simulink model "CloseLoop"  (R2024b)
settings: Solver=VariableStepAuto  StartTime=0.0  StopTime=10.0  FixedStep=0.001  RelTol=1e-7
values from neighbouring files (symbols this model uses):
  A = [0 0 0 1 0 0; 0 0 0 0 1 0; 0 0 0 0 0 1; 0 0 0 0 0 0; 0 0 0 0 0 0; 0 0 0 0 0 0]    [DefinedParameters.m]
  B = [0; 0; 0; 1; 1; 1]    [DefinedParameters.m]
  d = 0.0085    [DefinedParameters.m]
  D = J    (= 1.062e-08)    [DefinedParameters.m]
  Do = 0.0001    [DefinedParameters.m]
  F = 0.94    [DefinedParameters.m]
  g = 9.81    [DefinedParameters.m]
  h = 0.00515    [DefinedParameters.m]
  k = 71    [DefinedParameters.m]
  l = 0.03    [DefinedParameters.m]
  m = 0.0000354    (= 3.54e-05)    [DefinedParameters.m]
  r = 0.00485    [DefinedParameters.m]
libraries: simulink x12, matrix_library x2, slpidlib x1

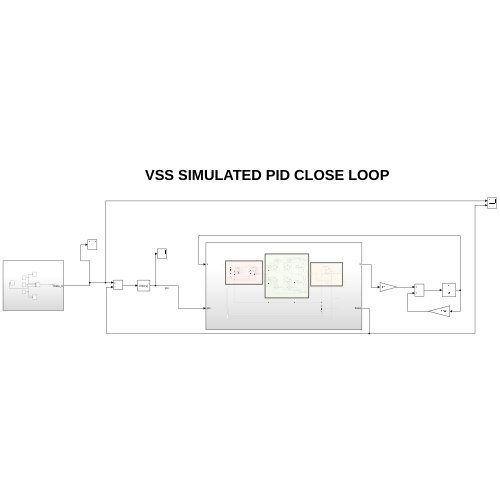
[thumbnail: Simulink's stored preview of the top-level diagram]
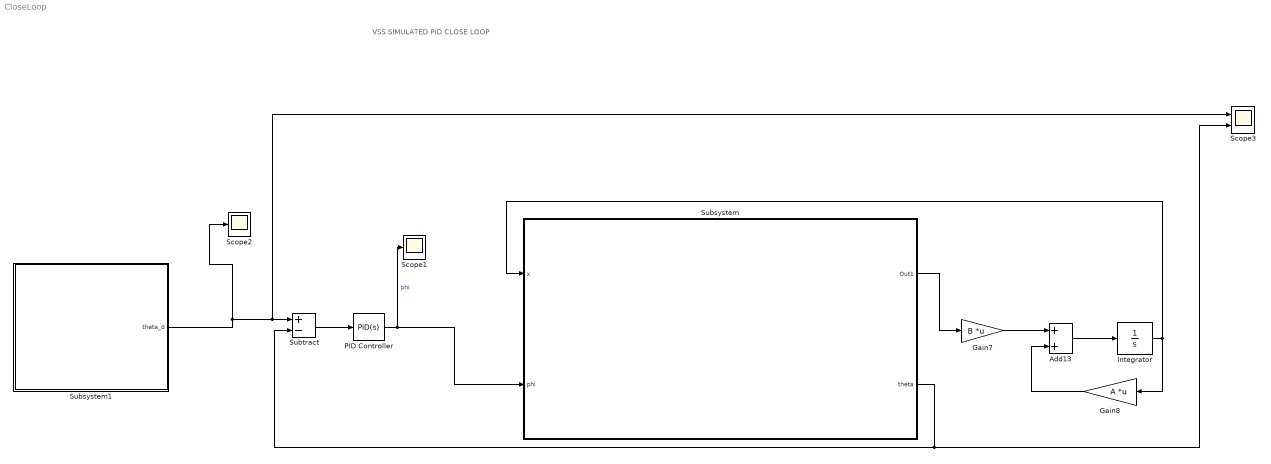
== system CloseLoop ==
  note: VSS SIMULATED PID CLOSE LOOP
  Add13 : Sum
  Gain7 : Gain  Gain=B  Multiplication=Matrix(K*u)
  Gain8 : Gain  Gain=A  Multiplication=Matrix(K*u)
  Integrator : Integrator  InitialCondition=[0;0;-1.6;0;0;0]
  PID Controller : slpidlib/PID Controller  Controller=PID  Form=Parallel  TimeDomain=Continuous-time  UseExternalTs=off  SampleTime=-1  IntegratorMethod=Forward Euler  FilterMethod=Forward Euler  ControllerParametersSource=internal  P=1  I=1.6  UseKiTs=off  D=0.5  UseExternalDerivativeSource=off  N=0  UseFilter=on  TunerSelectOption=Transfer Function Based (PID Tuner App)  InitialConditionSource=internal  InitialConditionForIntegrator=-1.7  InitialConditionForFilter=0  DifferentiatorICPrevScaledInput=0  ExternalReset=none  TrackingMode=off  Kt=1  LimitOutput=off  SatLimitsSource=internal  UpperSaturationLimit=inf  LowerSaturationLimit=-inf  LinearizeAsGain=on  AntiWindupMode=none  Kb=1  LimitIntegrator=off  UpperIntegratorSaturationLimit=inf  LowerIntegratorSaturationLimit=-inf  POutMin=[]  POutMax=[]  IOutMin=[]  IOutMax=[]  DOutMin=[]  DOutMax=[]  NOutMin=[]  NOutMax=[]  SumOutMin=[]  SumOutMax=[]  SaturationOutMin=[]  SaturationOutMax=[]  PParamMin=[]  PParamMax=[]  IParamMin=[]  IParamMax=[]  DParamMin=[]  DParamMax=[]  NParamMin=[]  NParamMax=[]  KbParamMin=[]  KbParamMax=[]  KtParamMin=[]  KtParamMax=[]  KbOutMin=[]  KbOutMax=[]  KtOutMin=[]  KtOutMax=[]  IntegratorOutMin=[]  IntegratorOutMax=[]  FilterOutMin=[]  FilterOutMax=[]  SumI1OutMin=[]  SumI1OutMax=[]  SumI2OutMin=[]  SumI2OutMax=[]  SumI3OutMin=[]  SumI3OutMax=[]  SumI4OutMin=[]  SumI4OutMax=[]  SumDOutMin=[]  SumDOutMax=[]  DifferentiatorOutMin=[]  DifferentiatorOutMax=[]  FilterDiffOutCoefMin=[]  FilterDiffOutCoefMax=[]  ReciprocalOutMin=[]  ReciprocalOutMax=[]  SumDenOutMin=[]  SumDenOutMax=[]  SumNumOutMin=[]  SumNumOutMax=[]  DivideOutMin=[]  DivideOutMax=[]  UdiffTsProdOutMin=[]  UdiffTsProdOutMax=[]  NTsProdOutMin=[]  NTsProdOutMax=[]  UintegralTsProdOutMin=[]  UintegralTsProdOutMax=[]  UngainTsProdOutMin=[]  UngainTsProdOutMax=[]  ClampingZeroOutDataTypeStr=Inherit: Inherit via back propagation  ClampingZeroOutMin=[]  ClampingZeroOutMax=[]  FilterDenConstantOutDataTypeStr=Inherit: Inherit via back propagation  FilterDenConstantOutMin=[]  FilterDenConstantOutMax=[]  PCopyOutDataTypeStr=Inherit: Inherit via back propagation  PCopyOutMin=[]  PCopyOutMax=[]  NCopyOutDataTypeStr=Inherit: Inherit via back propagation  NCopyOutMin=[]  NCopyOutMax=[]  IntegratorContinuousStateAttributes=''  IntegratorStateMustResolveToSignalObject=off  IntegratorRTWStateStorageClass=Auto  FilterContinuousStateAttributes=''  FilterStateMustResolveToSignalObject=off  FilterRTWStateStorageClass=Auto  ParallelPVariant=InternalParameters  IdealPVariant=Disabled  IVariant=InternalParameters  DVariant=InternalParameters  IntegratorVariant=Continuous  SatVariant=Disabled  AWVariant=Passthrough  PCopyVariant=Disabled  TRVariant=Disabled  FdbkBlocksVariant=Forward  IdealPFdbkVariant=Disabled  SatFdbkVariant=Disabled  DerivativeFilterVariant=ContFilter  NVariant=InternalParameters  NCopyVariant=Disabled  FilterICVariant=InternalICsFilter  IntegratorICVariant=InternalICs  ExternalResetVariant=Disabled  TRSumVariant=Passthrough  SumFdbkVariant=Disabled  SumVariant=Sum_PID  TsampFilterVariant=InternalTs  TsampNgainVariant=Passthrough  TsampIntegralVariant=Disabled_SignalSpec  ExternalSaturationOutDataTypeStr=Inherit: Same as second input  DerivativeSourceVariant=ErrorSignal  PreIntVariant=InternalPreInt
  Scope1 : Scope
  Scope2 : Scope
  Scope3 : Scope  NumInputPorts=2
  Subsystem : Subsystem
  Subsystem1 : Subsystem
  Subtract : Sum  Inputs=+-
  wires:
  Subtract/1 -> PID Controller/1
  Subsystem1/1(theta_d) -> Scope3/1, Subtract/1, Scope2/1
  PID Controller/1 -> Scope1/1, Subsystem/2(phi)  "phi"
  Subsystem/1(Out1) -> Gain7/1
  Gain8/1 -> Add13/2
  Integrator/1 -> Subsystem/1(x), Gain8/1
  Add13/1 -> Integrator/1
  Gain7/1 -> Add13/1
  Subsystem/2(theta) -> Subtract/2, Scope3/2

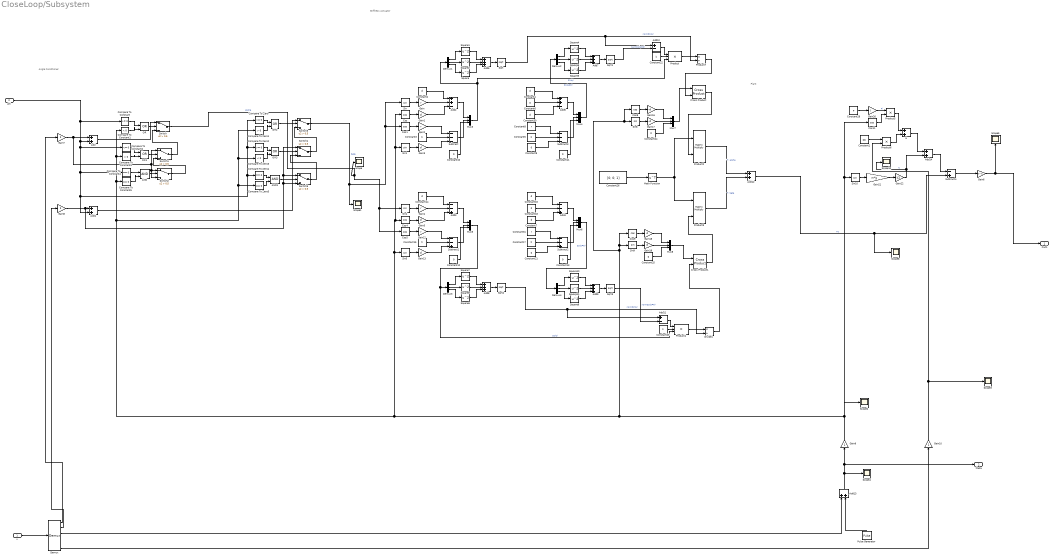
== system CloseLoop/Subsystem ==
  note: Plant
  note: Stiffness Actuator
  note: Angle Conditioner
  x : Inport
  phi : Inport  Port=2
  AND : Logic  IconShape=distinctive  AllPortsSameDT=off  OutDataTypeStr=boolean
  AND1 : Logic  IconShape=distinctive  AllPortsSameDT=off  OutDataTypeStr=boolean
  Add{,1,12..14} (5 alike) : Sum
  Add10 : Sum  Inputs=+-
  Add11 : Sum  Inputs=+-
  Add2 : Sum  Inputs=++-
  Add3 : Sum  Inputs=--+
  Add4 : Sum  Inputs=--+
  Add5 : Sum  Inputs=++-
  Add{6..9} (4 alike) : Sum  Inputs=+++
  Compare To Constant : simulink/Logic and Bit Operations/Compare To Constant  relop=>=  const=0  OutDataTypeStr=boolean
  Compare To Constant1 : simulink/Logic and Bit Operations/Compare To Constant  relop=<  const=0  OutDataTypeStr=boolean
  Compare To Constant2 : simulink/Logic and Bit Operations/Compare To Constant  relop=<=  const=0  OutDataTypeStr=boolean
  Compare To Constant3 : simulink/Logic and Bit Operations/Compare To Constant  relop=>  const=0  OutDataTypeStr=boolean
  Compare To Constant4 : simulink/Logic and Bit Operations/Compare To Constant  relop===  const=0  OutDataTypeStr=boolean
  Compare To Constant5 : simulink/Logic and Bit Operations/Compare To Constant  relop===  const=0  OutDataTypeStr=boolean
  Compare To Zero : simulink/Logic and Bit Operations/Compare To Zero  relop=<=  OutDataTypeStr=boolean
  Compare To Zero1 : simulink/Logic and Bit Operations/Compare To Zero  relop=>  OutDataTypeStr=boolean
  Compare To Zero2 : simulink/Logic and Bit Operations/Compare To Zero  relop=>=  OutDataTypeStr=boolean
  Compare To Zero3 : simulink/Logic and Bit Operations/Compare To Zero  relop=<  OutDataTypeStr=boolean
  Compare To Zero4 : simulink/Logic and Bit Operations/Compare To Zero  relop===  OutDataTypeStr=boolean
  Compare To Zero5 : simulink/Logic and Bit Operations/Compare To Zero  relop===  OutDataTypeStr=boolean
  Constant1 : Constant  Value=Do
  Constant{6,9..13,18,21,24..25} (10 alike) : Constant  Value=0
  Constant{2,4,7,14,16,30} (6 alike) : Constant  Value=d
  Constant{3,5,15,17} (4 alike) : Constant  Value=h
  Constant22 : Constant  Value=k
  Constant23 : Constant  Value=k
  Constant26 : Constant  Value=[0; 0; 1]
  Constant28 : Constant  Value=F
  Constant31 : Constant  Value=r
  Constant8 : Constant  Value=r
  Cos{,1,4..5,8..9,11} (7 alike) : Trigonometry  Operator=cos
  Cross Product : matrix_library/Cross Product
  Cross Product1 : matrix_library/Cross Product
  Demux : Demux  Outputs=6
  Demux{1..4} (4 alike) : Demux  Outputs=3
  Divide1 : Product  Inputs=*/
  Gain{,2,4,12} (4 alike) : Gain  Gain=r
  Gain{1,3,5,13,18..19} (6 alike) : Gain  Gain=d
  Gain{7..10} (4 alike) : Gain
  Gain16 : Gain  Gain=-d
  Gain17 : Gain  Gain=-d
  Gain21 : Gain  Gain=m*g
  Gain22 : Gain  Gain=l/2
  Gain26 : Gain  Gain=l
  Gain6 : Gain  Gain=D^-1
  H : Sum
  Math Function : Math  Operator=transpose
  Mux{3..8} (6 alike) : Mux  Inputs=3
  OR{,1..3} (4 alike) : Logic  Operator=OR  IconShape=distinctive  AllPortsSameDT=off  OutDataTypeStr=boolean
  Product : Product  Inputs=3
  Product1 : Product  Inputs=3
  Product2 : Product  Multiplication=Matrix(*)
  Product3 : Product  Multiplication=Matrix(*)
  Product5 : Product
  Product6 : Product
  Product7 : Product  Inputs=*/
  Pulse Generator : DiscretePulseGenerator  PulseType=Time based  Amplitude=0.02  Period=2.5  PulseWidth=0.5
  Scope{,1..5,8,10} (8 alike) : Scope
  Sin{,1,4..5,8..10} (7 alike) : Trigonometry
  Sqrt{,1..3} (4 alike) : Sqrt
  Square{,1..11} (12 alike) : Math  Operator=square
  Subtract : Sum  Inputs=---
  Subtract1 : Sum  Inputs=--+
  Subtract2 : Sum  Inputs=--+
  Subtract3 : Sum  Inputs=---
  Subtract4 : Sum  Inputs=-+
  Switch{,1..5} (6 alike) : Switch  Criteria=u2 > Threshold  Threshold=0.5  SaturateOnIntegerOverflow=off  InputSameDT=off
  Out1 : Outport
  theta : Outport  Port=2
  wires:
  x/1 -> Demux/1
  AND1/1 -> Switch5/2
  Switch5/1 -> Switch4/3
  Switch4/1 -> Switch3/3
  Add1/1 -> Switch3/1
  Gain8/1 -> Switch5/1, Switch4/1, Switch5/3, Add1/1
  Add/1 -> Switch/1
  Gain7/1 -> Add/1, Switch1/1, Switch2/3, Switch2/1
  OR3/1 -> Switch4/2
  OR2/1 -> Switch3/2
  Compare To Zero5/1 -> AND1/2
  Compare To Zero4/1 -> AND1/1
  Compare To Zero3/1 -> OR3/2
  Compare To Zero2/1 -> OR3/1
  Compare To Zero1/1 -> OR2/2
  Compare To Zero/1 -> OR2/1
  Switch2/1 -> Switch1/3
  AND/1 -> Switch2/2
  Compare To Constant5/1 -> AND/2
  Compare To Constant4/1 -> AND/1
  Constant16/1 -> Add4/1
  Sqrt3/1 -> Add11/2  "normS2(q=0)"
  Gain22/1 -> Scope10/1, Add14/2  "C"
  Product/1 -> Product7/1
  Switch/1 -> Scope/1, Sin4/1, Cos5/1  "alpha"
  Mux8/1 -> Cross Product1/1
  Gain4/1 -> Add3/2
  Add14/1 -> Subtract4/1
  Gain/1 -> Add2/2
  Demux3/3 -> Square6/1
  Product6/1 -> H/2
  Sin5/1 -> Gain13/1
  Math Function/1 -> Product3/1, Product2/1
  Cos11/1 -> Product5/2
  Product1/1 -> Divide1/1
  Add8/1 -> Sqrt2/1
  Constant6/1 -> Add5/2
  Constant21/1 -> Subtract2/3
  Constant26/1 -> Math Function/1
  Compare To Constant/1 -> OR/1
  Cos/1 -> Gain1/1
  Constant31/1 -> Subtract2/1
  Product3/1 -> Add12/2  "T, beta"
  Constant4/1 -> Add5/1
  Constant2/1 -> Add2/1
  Product2/1 -> Add12/1  "T, alpha"
  Subtract/1 -> Mux3/2
  Product5/1 -> H/1
  H/1 -> Add14/1
  Demux2/2 -> Square5/1
  Sin10/1 -> Gain21/1
  Gain1/1 -> Add2/3
  Cross Product1/1 -> Product3/2
  Mux6/1 -> Demux4/1  "S2(q=0)"
  Constant13/1 -> Mux6/3
  Demux3/1 -> Square7/1
  Constant22/1 -> Product/2
  Demux3/2 -> Square8/1
  Mux7/1 -> Cross Product/1
  Constant8/1 -> Subtract3/1
  Switch3/1 -> Scope1/1, Sin/1, Cos1/1  "beta"
  Cos5/1 -> Gain12/1
  Subtract1/1 -> Mux5/2
  Square8/1 -> Add8/2
  Gain13/1 -> Subtract1/3
  Cos9/1 -> Gain18/1
  Add11/1 -> Product1/1
  Square1/1 -> Add6/1
  Gain2/1 -> Subtract/1
  Add3/1 -> Mux5/1
  Sqrt1/1 -> Add10/2  "normS1(q=0)"
  Constant5/1 -> Subtract3/2
  Sin4/1 -> Gain4/1
  Square6/1 -> Add8/3
  Compare To Constant2/1 -> OR1/1
  Constant14/1 -> Add3/1
  Constant7/1 -> Add4/3
  Gain5/1 -> Add3/3
  Demux2/1 -> Square4/1
  Sin/1 -> Gain/1
  Constant25/1 -> Mux8/3
  Square9/1 -> Add9/3
  Square2/1 -> Add6/2
  Sin8/1 -> Gain17/1
  Square3/1 -> Add7/3
  Square4/1 -> Add7/1
  Gain16/1 -> Mux7/1
  Mux5/1 -> Demux3/1, Product1/3  "S2(q)"
  Add10/1 -> Product/1
  Compare To Constant3/1 -> OR1/2
  Sin9/1 -> Gain19/1
  Sqrt2/1 -> Divide1/2, Add11/1  "normS2(q)"
  Gain10/1 -> Product6/2, Scope3/1
  Constant3/1 -> Subtract/2
  Mux3/1 -> Demux1/1, Product/3  "S1(q)"
  Constant10/1 -> Mux3/3
  Cos8/1 -> Gain16/1
  Gain6/1 -> Out1/1, Scope5/1
  Sin1/1 -> Gain3/1
  Sqrt/1 -> Add10/1, Product7/2  "normS1(q)"
  Demux4/1 -> Square10/1
  Constant17/1 -> Subtract2/2
  Demux1/2 -> Square2/1
  Demux4/2 -> Square11/1
  Divide1/1 -> Cross Product1/2
  Cos1/1 -> Gain2/1
  Add6/1 -> Sqrt/1
  phi/1 -> Compare To Constant/1, Add/2, Compare To Constant2/1, Compare To Constant4/1, Compare To Zero4/1, Compare To Zero2/1, Compare To Zero/1, Add1/2
  Constant30/1 -> Add5/3
  Cos4/1 -> Gain5/1
  Constant28/1 -> Gain26/1
  Mux4/1 -> Demux2/1  "S1(q=0)"
  Constant12/1 -> Mux5/3
  Add2/1 -> Mux3/1
  Gain9/1 -> Compare To Constant1/1, Compare To Constant3/1, Compare To Constant5/1, Compare To Zero5/1, Compare To Zero3/1, Compare To Zero1/1, Sin5/1, Cos4/1, Sin1/1, Cos/1, Cos9/1, Sin9/1, Sin8/1, Cos8/1, Sin10/1, Cos11/1, Scope2/1
  Gain18/1 -> Mux8/1
  Square7/1 -> Add8/1
  Gain26/1 -> Product5/1  "Fl"
  Switch1/1 -> Switch/3
  Gain21/1 -> Gain22/1
  OR1/1 -> Switch1/2
  Demux1/1 -> Square1/1
  Square5/1 -> Add7/2
  Constant15/1 -> Subtract1/2
  Subtract4/1 -> Gain6/1
  Gain3/1 -> Subtract/3
  Add12/1 -> Scope8/1, Subtract4/2  "To"
  Subtract3/1 -> Mux4/2
  Gain17/1 -> Mux7/2
  Compare To Constant1/1 -> OR/2
  Add7/1 -> Sqrt1/1
  Constant24/1 -> Mux7/3
  Product7/1 -> Cross Product/2
  Constant1/1 -> Product6/1
  Add9/1 -> Sqrt3/1
  Gain19/1 -> Mux8/2
  Square10/1 -> Add9/1
  Subtract2/1 -> Mux6/2
  Square11/1 -> Add9/2
  Add4/1 -> Mux6/1
  OR/1 -> Switch/2
  Gain12/1 -> Subtract1/1
  Square/1 -> Add6/3
  Constant11/1 -> Mux4/3
  Constant23/1 -> Product1/2
  Demux1/3 -> Square/1
  Add5/1 -> Mux4/1
  Demux4/3 -> Square9/1
  Cross Product/1 -> Product2/2
  Constant9/1 -> Subtract3/3
  Demux2/3 -> Square3/1
  Constant18/1 -> Add4/2
  Add13/1 -> theta/1, Gain9/1, Scope4/1
  Pulse Generator/1 -> Add13/2
  Demux/3 -> Add13/1
  Demux/6 -> Gain10/1
  Demux/1 -> Gain7/1
  Demux/2 -> Gain8/1

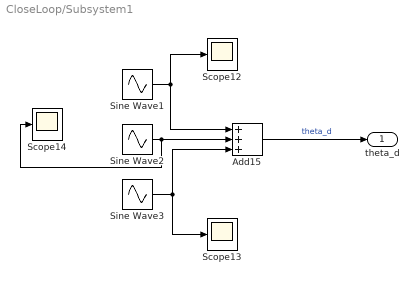
== system CloseLoop/Subsystem1 ==
  Add15 : Sum  Inputs=+++
  Scope12 : Scope
  Scope13 : Scope
  Scope14 : Scope
  Sine Wave1 : Sin  Amplitude=0.1  Frequency=2  Phase=pi  SampleTime=0
  Sine Wave2 : Sin  Amplitude=0.03  Frequency=4  Phase=pi  SampleTime=0
  Sine Wave3 : Sin  Amplitude=0.015  Frequency=6  Phase=pi  SampleTime=0
  theta_d : Outport
  wires:
  Sine Wave1/1 -> Scope12/1, Add15/1
  Sine Wave3/1 -> Add15/3, Scope13/1
  Sine Wave2/1 -> Add15/2, Scope14/1
  Add15/1 -> theta_d/1  "theta_d"
